simulink model "CT_POI"  (R2022a)
settings: Solver=ode45  StartTime=0.0  StopTime=101.01e-3  RelTol=1e-3  EnableMultiTasking=on
undefined symbols (not defined in the file): DiscIntNeverNeededParam, ln
libraries: commseqgen3 x2, commutil2 x2, dspstat3 x2, dsparch4 x1
settings Model: SimulationMode=accelerator  Creator=Home  LastModifiedBy=Anastasia
settings SolverCC: AlgebraicLoopSolver=TrustRegion
settings DataIOCC: LimitDataPoints=on  SaveFormat=Array  SignalLoggingSaveFormat=ModelDataLogs  ReturnWorkspaceOutputs=off
settings OptimizationCC: ExpressionDepthLimit=2147483647  InitFltsAndDblsToZero=on  LifeSpan=inf
settings DebuggingCC: SaveWithParameterizedLinksMsg=none  UnderspecifiedInitializationDetection=Classic  MergeDetectMultiDrivingBlocksExec=none  SignalResolutionControl=TryResolveAllWithWarning  SolverPrmCheckMsg=warning  MultiTaskDSMMsg=warning  MultiTaskCondExecSysMsg=none  FcnCallInpInsideContextMsg=warning  UnconnectedInputMsg=warning  UnconnectedOutputMsg=warning  UnconnectedLineMsg=warning  StateNameClashWarn=warning  SFUnexpectedBacktrackingDiag=warning  SFNoUnconditionalDefaultTransitionDiag=warning  SFExecutionAtInitializationDiag=none  SFMachineParentedDataDiag=warning  ArithmeticOperatorsInVariantConditions=warning
settings HardwareCC: ProdBitPerPointer=32  ProdBitPerSizeT=32  ProdBitPerPtrDiffT=32  ProdLargestAtomicFloat=None  ProdIntDivRoundTo=Undefined  ProdEndianess=Unspecified  ProdWordSize=32  ProdHWDeviceType=32-bit Generic
settings ModelReferenceCC: PropagateSignalLabelsOutOfModel=off
settings CodeAppCC: StateflowObjectComments=on
settings GRTTargetCC: TargetFcnLib=ansi_tfl_tmw.mat  TargetLangStandard=C89/C90 (ANSI)  CombineOutputUpdateFcns=off  GRTInterface=on
settings ConfigComp: CovMetricSettings=dw  CovSaveCumulativeToWorkspaceVar=on  CovSaveSingleToWorkspaceVar=on

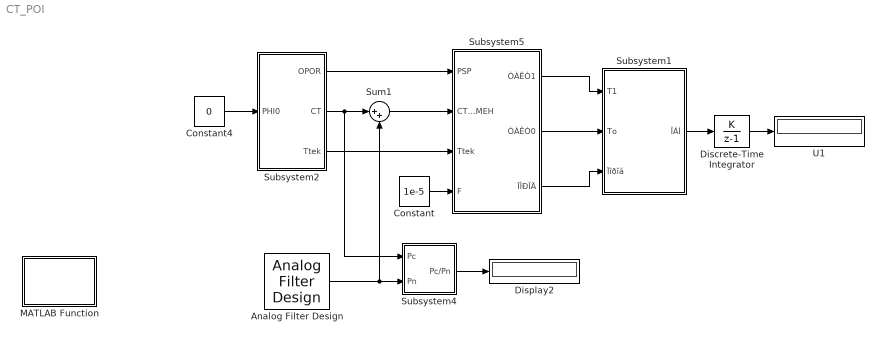
== system CT_POI ==
  Analog Filter Design : dsparch4/Analog Filter Design  method=Chebyshev II  filttype=Bandpass  N=10  Wlo=2*pi*2e6  Whi=2*pi*3e6  Rp=3  Rs=40
  Constant : Constant  Value=1e-5
  Constant4 : Constant  Value=0  VectorParams1D=off  SampleTime=1e-3
  Discrete-Time Integrator : DiscreteIntegrator  IntegratorMethod=Accumulation: Forward Euler  gainval=1/100  SampleTime=1e-3  ICPrevOutput=DiscIntNeverNeededParam  ICPrevScaledInput=DiscIntNeverNeededParam
  Display2 : Display
  MATLAB Function : MATLAB Function  TreatAsAtomicUnit=on
  Subsystem1 : Subsystem
  Subsystem2 : Subsystem
  Subsystem4 : Subsystem
  Subsystem5 : Subsystem
  Sum1 : Sum  Inputs=|++
  U1 : Display
  wires:
  Subsystem2/1(OPOR) -> Subsystem5/1(PSP)
  Constant4/1 -> Subsystem2/1(PHI0)
  Subsystem2/3(Ttek) -> Subsystem5/3(Ttek)
  Analog Filter Design/1 -> Subsystem4/2(Pn), Sum1/2
  ? -> Analog Filter Design/1
  Subsystem2/2(CT) -> Sum1/1, Subsystem4/1(Pc)
  Sum1/1 -> Subsystem5/2(CT+POMEH)
  Subsystem4/1(Pc/Pn) -> Display2/1
  Constant/1 -> Subsystem5/4(F)
  Subsystem5/1(ÒÀÊÒ1) -> Subsystem1/1(T1)
  Subsystem5/2(ÒÀÊÒ0) -> Subsystem1/2(To)
  Subsystem5/3(ÏÎÐÎÃ) -> Subsystem1/3(Ïîðîã)
  Discrete-Time Integrator/1 -> U1/1
  Subsystem1/1(ÎÁÍ) -> Discrete-Time Integrator/1

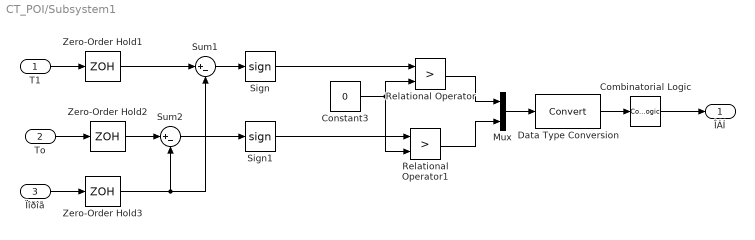
== system CT_POI/Subsystem1 ==
  T1 : Inport
  To : Inport  Port=2
  Ïîðîã : Inport  Port=3
  Combinatorial Logic : CombinatorialLogic  TruthTable=[0;0;1;0]
  Constant3 : Constant  Value=0  SampleTime=-1
  Data Type Conversion : DataTypeConversion  SaturateOnIntegerOverflow=off  RndMeth=Floor
  Mux : Mux  Inputs=2
  Relational Operator : RelationalOperator  Operator=>  OutDataTypeStr=boolean  InputSameDT=off
  Relational Operator1 : RelationalOperator  Operator=>  OutDataTypeStr=boolean  InputSameDT=off
  Sign : Signum
  Sign1 : Signum
  Sum1 : Sum  Inputs=|+-
  Sum2 : Sum  Inputs=|+-
  Zero-Order Hold1 : ZeroOrderHold  SampleTime=1e-3
  Zero-Order Hold2 : ZeroOrderHold  SampleTime=1e-3
  Zero-Order Hold3 : ZeroOrderHold  SampleTime=1e-3
  ÎÁÍ : Outport
  wires:
  Sum2/1 -> Sign1/1
  Zero-Order Hold1/1 -> Sum1/1
  Zero-Order Hold2/1 -> Sum2/1
  Zero-Order Hold3/1 -> Sum2/2, Sum1/2
  Sum1/1 -> Sign/1
  T1/1 -> Zero-Order Hold1/1
  To/1 -> Zero-Order Hold2/1
  Ïîðîã/1 -> Zero-Order Hold3/1
  Sign/1 -> Relational Operator/1
  Sign1/1 -> Relational Operator1/1
  Constant3/1 -> Relational Operator/2, Relational Operator1/2
  Relational Operator/1 -> Mux/1
  Relational Operator1/1 -> Mux/2
  Data Type Conversion/1 -> Combinatorial Logic/1
  Mux/1 -> Data Type Conversion/1
  Combinatorial Logic/1 -> ÎÁÍ/1

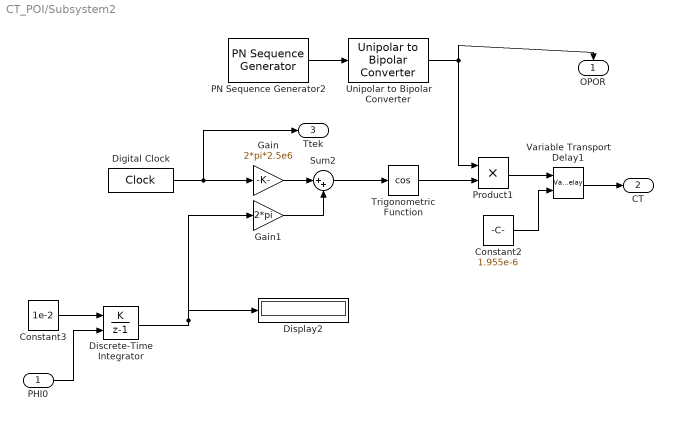
== system CT_POI/Subsystem2 ==
  PHI0 : Inport
  Constant2 : Constant  Value=1.955e-6
  Constant3 : Constant  Value=1e-2  SampleTime=1e-3
  Digital Clock : DigitalClock  SampleTime=1.955e-7
  Discrete-Time Integrator : DiscreteIntegrator  IntegratorMethod=Accumulation: Forward Euler  gainval=1  InitialConditionSource=external  SampleTime=1e-3  ICPrevOutput=DiscIntNeverNeededParam  ICPrevScaledInput=DiscIntNeverNeededParam
  Display2 : Display
  Gain : Gain  Gain=2*pi*2.5e6
  Gain1 : Gain  Gain=2*pi
  PN Sequence Generator2 : commseqgen3/PN Sequence Generator  poly=[1 0 0 0 0 1 0 0 0 1]  ini_sta=[1 1 1 1 1 1 1 1 1]  outBitMaskSource=Dialog parameter  shift=0  outVarSiz=off  maxOutSizeMode=Dialog parameter  maxOutSize=[10 1]  Ts=1.955e-6  sampPerFrame=1  reset=off  bitPackedOutputs=off  outDataType=boolean  numPackedBits=8  bitPackDataSigned=off  bitPackedOutDType=double
  Product1 : Product  RndMeth=Zero
  Sum2 : Sum  Inputs=|++
  Trigonometric Function : Trigonometry  Operator=cos
  Unipolar to Bipolar Converter : commutil2/Unipolar to Bipolar Converter  M=2  polarity=Positive  dataType=double
  Variable Transport Delay1 : VariableTransportDelay  MaximumDelay=511
  OPOR : Outport
  CT : Outport  Port=2
  Ttek : Outport  Port=3
  wires:
  Unipolar to Bipolar Converter/1 -> Product1/1, OPOR/1
  PN Sequence Generator2/1 -> Unipolar to Bipolar Converter/1
  Digital Clock/1 -> Gain/1, Ttek/1
  Sum2/1 -> Trigonometric Function/1
  Gain/1 -> Sum2/1
  Gain1/1 -> Sum2/2
  Trigonometric Function/1 -> Product1/2
  Constant2/1 -> Variable Transport Delay1/2
  Product1/1 -> Variable Transport Delay1/1
  Variable Transport Delay1/1 -> CT/1
  Constant3/1 -> Discrete-Time Integrator/1
  PHI0/1 -> Discrete-Time Integrator/2
  Discrete-Time Integrator/1 -> Gain1/1, Display2/1

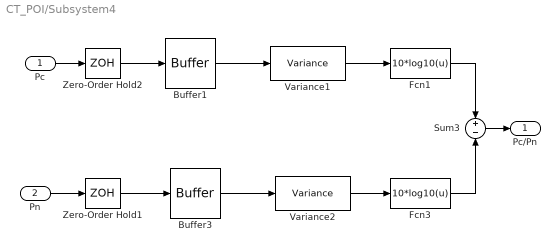
== system CT_POI/Subsystem4 ==
  Pc : Inport
  Pn : Inport  Port=2
  Buffer1 : Buffer  N=511*5
  Buffer3 : Buffer  N=511*5
  Fcn1 : Fcn  Expr=10*log10(u)
  Fcn3 : Fcn  Expr=10*log10(u)
  Sum3 : Sum  Inputs=+-
  Variance1 : dspstat3/Variance  run=off  InputProcessing=Columns as channels (frame based)  reset_popup=None  directionMode=Each column  dimension=1  roiEnable=off  roiType=Rectangles  roiPortion=Entire ROI  roiOutput=Individual statistics for each ROI  roiFlag=off  roundingMode=Floor  overflowMode=off
  Variance2 : dspstat3/Variance  run=off  InputProcessing=Columns as channels (frame based)  reset_popup=None  directionMode=Each column  dimension=1  roiEnable=off  roiType=Rectangles  roiPortion=Entire ROI  roiOutput=Individual statistics for each ROI  roiFlag=off  roundingMode=Floor  overflowMode=off
  Zero-Order Hold1 : ZeroOrderHold  SampleTime=1.955e-7
  Zero-Order Hold2 : ZeroOrderHold  SampleTime=1.955e-7
  Pc/Pn : Outport
  wires:
  Zero-Order Hold1/1 -> Buffer3/1
  Buffer3/1 -> Variance2/1
  Variance2/1 -> Fcn3/1
  Fcn3/1 -> Sum3/2
  Zero-Order Hold2/1 -> Buffer1/1
  Buffer1/1 -> Variance1/1
  Variance1/1 -> Fcn1/1
  Fcn1/1 -> Sum3/1
  Pc/1 -> Zero-Order Hold2/1
  Pn/1 -> Zero-Order Hold1/1
  Sum3/1 -> Pc/Pn/1

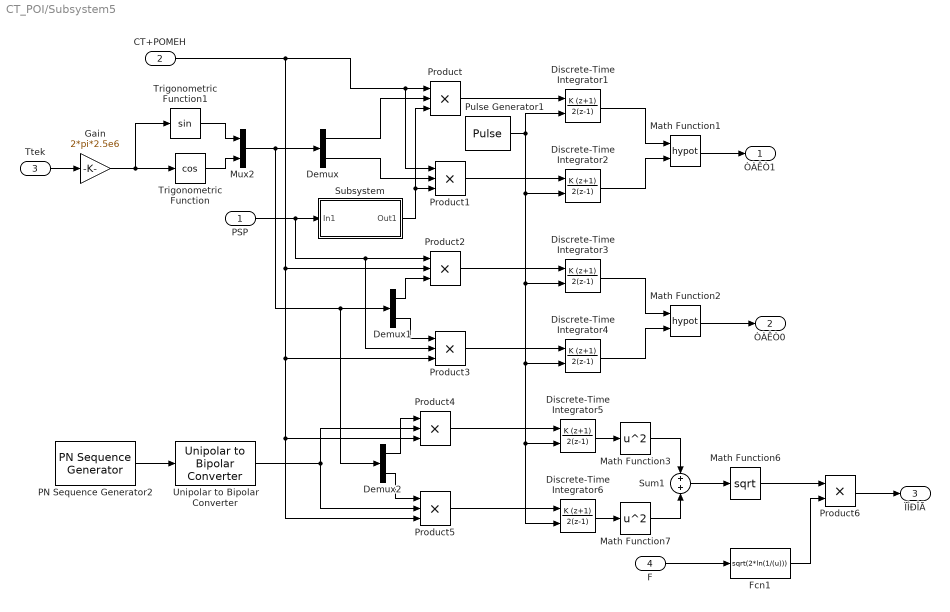
== system CT_POI/Subsystem5 ==
  PSP : Inport
  CT+POMEH : Inport  Port=2
  Ttek : Inport  Port=3
  F : Inport  Port=4
  Demux : Demux  Outputs=2
  Demux1 : Demux  Outputs=2
  Demux2 : Demux  Outputs=2
  Discrete-Time Integrator{1..6} (6 alike) : DiscreteIntegrator  IntegratorMethod=Accumulation: Trapezoidal  gainval=1/(511*10)  ExternalReset=falling  SampleTime=1.955e-7  ICPrevOutput=DiscIntNeverNeededParam  ICPrevScaledInput=DiscIntNeverNeededParam
  Fcn1 : Fcn  Expr=sqrt(2*ln(1/(u)))
  Gain : Gain  Gain=2*pi*2.5e6
  Math Function1 : Math  Operator=hypot  SignedPower=on
  Math Function2 : Math  Operator=hypot  SignedPower=on
  Math Function3 : Math  Operator=square  SignedPower=on
  Math Function6 : Math  Operator=sqrt  SignedPower=on
  Math Function7 : Math  Operator=square  SignedPower=on
  Mux2 : Mux  Inputs=2
  PN Sequence Generator2 : commseqgen3/PN Sequence Generator  poly=[9 4 0]  ini_sta=[1 0 1 1 1 0 1 1 1]  outBitMaskSource=Dialog parameter  shift=0  outVarSiz=off  maxOutSizeMode=Dialog parameter  maxOutSize=[10 1]  Ts=1.955e-6  sampPerFrame=1  reset=off  bitPackedOutputs=off  outDataType=boolean  numPackedBits=8  bitPackDataSigned=off  bitPackedOutDType=double
  Product{,1..5} (6 alike) : Product  Inputs=3  RndMeth=Zero
  Product6 : Product  RndMeth=Zero
  Pulse Generator1 : DiscretePulseGenerator  PulseType=Time based  Period=1e-3  PulseWidth=50  PhaseDelay=0.5e-3
  Subsystem : Subsystem
  Sum1 : Sum
  Trigonometric Function : Trigonometry  Operator=cos
  Trigonometric Function1 : Trigonometry
  Unipolar to Bipolar Converter : commutil2/Unipolar to Bipolar Converter  M=2  polarity=Positive  dataType=double
  ÒÀÊÒ1 : Outport
  ÒÀÊÒ0 : Outport  Port=2
  ÏÎÐÎÃ : Outport  Port=3
  wires:
  Mux2/1 -> Demux/1, Demux1/1, Demux2/1
  Pulse Generator1/1 -> Discrete-Time Integrator1/2, Discrete-Time Integrator2/2, Discrete-Time Integrator3/2, Discrete-Time Integrator4/2, Discrete-Time Integrator5/2, Discrete-Time Integrator6/2
  Product/1 -> Discrete-Time Integrator1/1
  Demux/1 -> Product/2
  Product1/1 -> Discrete-Time Integrator2/1
  Demux/2 -> Product1/2
  CT+POMEH/1 -> Product/1, Product1/1, Product2/2, Product3/3, Product4/3, Product5/3
  Discrete-Time Integrator1/1 -> Math Function1/1
  Discrete-Time Integrator2/1 -> Math Function1/2
  PSP/1 -> Subsystem/1(In1), Product2/1, Product3/2
  Subsystem/1(Out1) -> Product/3, Product1/3
  Math Function1/1 -> ÒÀÊÒ1/1
  Ttek/1 -> Gain/1
  Gain/1 -> Trigonometric Function/1, Trigonometric Function1/1
  Trigonometric Function1/1 -> Mux2/1
  Trigonometric Function/1 -> Mux2/2
  Product2/1 -> Discrete-Time Integrator3/1
  Product3/1 -> Discrete-Time Integrator4/1
  Discrete-Time Integrator3/1 -> Math Function2/1
  Discrete-Time Integrator4/1 -> Math Function2/2
  Math Function2/1 -> ÒÀÊÒ0/1
  Demux1/1 -> Product2/3
  Demux1/2 -> Product3/1
  Product4/1 -> Discrete-Time Integrator5/1
  Product5/1 -> Discrete-Time Integrator6/1
  Discrete-Time Integrator5/1 -> Math Function3/1
  Discrete-Time Integrator6/1 -> Math Function7/1
  F/1 -> Fcn1/1
  Product6/1 -> ÏÎÐÎÃ/1
  Sum1/1 -> Math Function6/1
  Fcn1/1 -> Product6/2
  Math Function6/1 -> Product6/1
  Math Function3/1 -> Sum1/1
  Math Function7/1 -> Sum1/2
  PN Sequence Generator2/1 -> Unipolar to Bipolar Converter/1
  Unipolar to Bipolar Converter/1 -> Product5/2, Product4/2
  Demux2/1 -> Product4/1
  Demux2/2 -> Product5/1

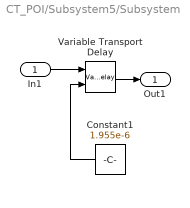
== system CT_POI/Subsystem5/Subsystem ==
  In1 : Inport
  Constant1 : Constant  Value=1.955e-6  SampleTime=-1
  Variable Transport Delay : VariableTransportDelay  VariableDelayType=Variable transport delay  MaximumDelay=2
  Out1 : Outport
  wires:
  Constant1/1 -> Variable Transport Delay/2
  In1/1 -> Variable Transport Delay/1
  Variable Transport Delay/1 -> Out1/1

== matlab function CT_POI/MATLAB Function ==
function rand
u = randn;
